simulink model "formation_planner_exp_cs_old"  (R2022b)
settings: Solver=ode5  StartTime=0.0  StopTime=80  FixedStep=1/1000  RelTol=1e-3
PreLoadFcn:
  | mbxruntime.callbacks.PreLoadFcn(bdroot);
PostLoadFcn:
  | mbxruntime.callbacks.PostLoadFcn(bdroot);
InitFcn:
  | mbxruntime.callbacks.InitFcn(bdroot);
StartFcn:
  | mbxruntime.callbacks.StartFcn(bdroot);
StopFcn:
  | mbxruntime.callbacks.StopFcn(bdroot);
model workspace (MAT data in the model file):
  mbox_table : object (value not decoded)
  model_closed = 0
  sim_status = 0
values from neighbouring files (symbols this model uses):
  c_factor = 43.75    [emplanner_init.m]
  car1_s = -10    [emplanner_init.m]
  car2_s = -20    [emplanner_init.m]
  cf = -175016    [emplanner_init.m]
  cr = -130634    [emplanner_init.m]
  KD_PID_distance = 0.0    (= 0)    [emplanner_init.m]
  KD_PID_speed = 0    [emplanner_init.m]
  KI_PID_distance = 0.0    (= 0)    [emplanner_init.m]
  KI_PID_speed = 0    [emplanner_init.m]
  KP_PID_distance = 0.5    [emplanner_init.m]
  KP_PID_speed = 1.8    [emplanner_init.m]
  la = 1.265    [emplanner_init.m]
  lb = 2.947-1.265    (= 1.682)    [emplanner_init.m]
  leader_global_kappa = global_kappa    [kappa.m]    (also in leader_global_path.mat = [0 0 0 0 0 0 0 0 0 0 0 0 ... (801 elements, 801x1)])
  leader_global_path_x = x_orgin.Data    [kappa.m]    (also in leader_global_path.mat = [2.22044604925e-16 0.999382255067 1.99750536558 2.9943522493)
  leader_global_path_y = y.Data    [kappa.m]    (also in leader_global_path.mat = [2 2 2 2 2 2 2 2 2 2 2 2 ... (801 elements, 801x1)])
  leader_global_yaw = yaw.Data    [kappa.m]    (also in leader_global_path.mat = [0 0 0 0 0 0 0 0 0 0 0 0 ... (801 elements, 801x1)])
  LQR_K1 = k(:,1)'    [emplanner_init.m]
  LQR_K2 = k(:,2)'    [emplanner_init.m]
  LQR_K3 = k(:,3)'    [emplanner_init.m]
  LQR_K4 = k(:,4)'    [emplanner_init.m]
  m = 2020    [emplanner_init.m]
  rack_displacement = [-39.14 , -37.2 , -35.29 , -33.43 , -31.6 , -29.81 , -28.06 , -26.34 , -24.66 ,      -23.01 , -21.38 , -19.79 , -18.23 , -16.69 , -15.18 , -13.7 , -12.23 , -10.8 , -9.38 , -7.98 ,     -6.61 , -5.25 , -3.91 , -2.59 , -1.29 , 0 , 1.27 , 2.54 , 3.78 , 5.02 , 6.24 , 7.46 , 8.66 ,      9.86 , 11.05 , 12.24 , 13.41 , 14.59 , 15.76 , 16.92 , 18.09 , 19.25 , 20.42 , 21.59 , 22.76 ,      23.93 , 25.11 , 26 ...(+26 chars)    [emplanner_init.m]
  right_wheel_ground = [-70 ,-67.2 , -64.4 , -61.6 , -58.8 , -56 , -53.2 , -50.4 , -47.6 , -44.8 , -42 ,      -39.2 , -36.4 , -33.6 , -30.8 , -28 , -25.2 , -22.4 , -19.6 , -16.8 , -14 , -11.2 , -8.4 , -5.6 ,      -2.8 , 0 , 2.8 , 5.6 , 8.4 , 11.2 , 14 , 16.8 , 19.6 , 22.4 , 25.2 , 28 , 30.8 , 33.6 , 36.4 ,      39.2 , 42 , 44.8 , 47.6 , 50.4 , 53.2 , 56 , 58.8 , 61.6 , 64.4 , 67.2 , 70 ]    [emplanner_init.m]
  vx_break_point = zeros(1,5000)    [emplanner_init.m]
undefined symbols (not defined in the file or in its folder): aubr, car1_global_kappa, car1_global_path_x, car1_global_path_y, car1_global_yaw, car2_global_kappa, car2_global_path_x, car2_global_path_y, car2_global_yaw, DiscIntNeverNeededParam, tablebr, vubr, warningInitialVelocity, x0
libraries: PreScanSimulinkLibrary x65, simulink x19, simulink_extras x14, Solver_SF x2
(part 10 of 31)

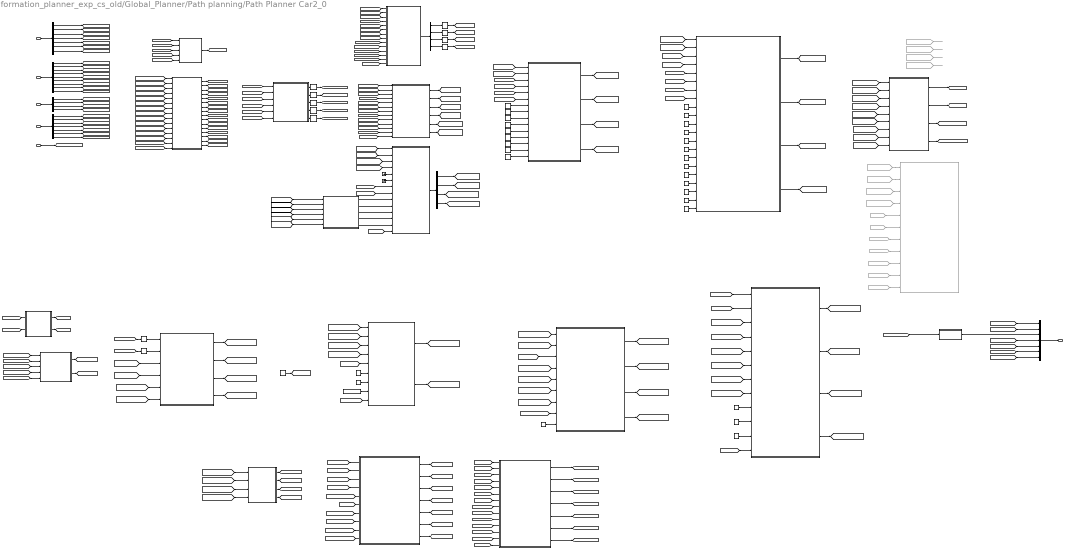
== system formation_planner_exp_cs_old/Global_Planner/Path planning/Path Planner Car2_0 ==
  referenceline info : Inport
  location info : Inport  Port=2
  perception info : Inport  Port=3
  pre_planning info : Inport  Port=4
  current time : Inport  Port=5
  Bus Creator : BusCreator  Inputs=7
  Bus Selector : BusSelector  OutputSignals=referenceline_x,referenceline_y,referenceline_heading,referenceline_kappa,origin_match_point_index,origin_x,origin_y
  Bus Selector1 : BusSelector  OutputSignals=host_x,host_y,host_heading_xy,host_vx,host_vy,host_yawrate,host_speed,host_ax,host_ay
  Bus Selector2 : BusSelector  OutputSignals=obs_x_set_gcs,obs_y_set_gcs,obs_velocity_set_gcs,obs_heading_set_gcs
  Bus Selector3 : BusSelector  OutputSignals=trajectory_x_gcs,trajectory_y_gcs,trajectory_heading_gcs,trajectory_kappa_gcs,trajectory_speed_gcs,trajectory_accel_gcs,trajectory_time_gcs
  Bus Selector4 : BusSelector  OutputSignals=s_set,l_set,dl_set,ddl_set
  Bus Selector5 : BusSelector  OutputSignals=s_set,l_set,s_dot_set,l_dot_set
  Cartesian2Frenet : Subsystem
  Cartesian2Frenet1 : Subsystem
  Constant : Constant  Value=1e6
  Constant1 : Constant  Value=2000
  Constant10 : Constant  Value=0.1
  Constant11 : Constant  Value=0.02
  Constant12 : Constant  Value=5
  Constant13 : Constant  Value=25000
  Constant14 : Constant  Value=50
  Constant15 : Constant  Value=20
  Constant16 : Constant  Value=50
  Constant{7,17..19} (4 alike) : Constant  Value=15
  Constant2 : Constant  Value=2
  Constant20 : Constant  Value=3
  Constant21 : Constant  Value=3
  Constant22 : Constant  Value=1.63
  Constant23 : Constant  Value=11
  Constant24 : Constant  Value=4000
  Constant25 : Constant  Value=100
  Constant26 : Constant  Value=10000000
  Constant27 : Constant  Value=0.2*9.8
  Constant28 : Constant  Value=50
  Constant29 : Constant  Value=500
  Constant3 : Constant  Value=3
  Constant4 : Constant  Value=10
  Constant5 : Constant  Value=11
  Constant6 : Constant  Value=4
  Constant8 : Constant
  Constant9 : Constant  Value=10
  Delay : Delay  DelayLength=1
  Delay1 : Delay  DelayLength=1
  Frenet2Cartesian task : MATLAB Function  TreatAsAtomicUnit=on
  From103 : From  Commented=on  GotoTag=dp_path_s_final
  From109 : From  Commented=on  GotoTag=dp_path_l_final
  From116 : From  Commented=on  GotoTag=dp_path_dl_final
  From117 : From  Commented=on  GotoTag=dp_path_ddl_final
  From120 : From  Commented=on  GotoTag=dp_path_s_final
  From124 : From  Commented=on  GotoTag=dp_path_l_final
  From125 : From  Commented=on  GotoTag=l_min
  From126 : From  Commented=on  GotoTag=l_max
  From129 : From  Commented=on  GotoTag=plan_start_l
  From130 : From  Commented=on  GotoTag=plan_start_dl
  From131 : From  Commented=on  GotoTag=plan_start_s
  From132 : From  Commented=on  GotoTag=static_obs_s_set
  From133 : From  Commented=on  GotoTag=static_obs_l_set
  From91 : From  Commented=on  GotoTag=qp_path_s_final
  From92 : From  Commented=on  GotoTag=qp_path_l_final
  Ground : Ground
  Ground1 : Ground
  MATLAB Function : MATLAB Function  TreatAsAtomicUnit=on
  MATLAB Function1 : MATLAB Function  TreatAsAtomicUnit=on
  MATLAB Function2 : MATLAB Function  TreatAsAtomicUnit=on
  Selector{1..9} (9 alike) : Selector  InputPortWidth=128  IndexOptions=Index vector (dialog)  Indices=1  OutputSizes=1
  calc path length and map between point and s1 : MATLAB Function  TreatAsAtomicUnit=on
  calc plan start info and stitch trajectory : MATLAB Function  TreatAsAtomicUnit=on
  calc speed planning start condition : MATLAB Function  TreatAsAtomicUnit=on
  generate convex space : MATLAB Function  TreatAsAtomicUnit=on
  generate st graph : MATLAB Function  TreatAsAtomicUnit=on
  genrate index to s : MATLAB Function  TreatAsAtomicUnit=on
  increase st point count : MATLAB Function  TreatAsAtomicUnit=on
  obs : Subsystem
  path and speed merge : MATLAB Function  TreatAsAtomicUnit=on
  path decision task : Subsystem
  path planning task : Subsystem
  plot : MATLAB Function  Commented=on  TreatAsAtomicUnit=on
  speed decision with dynamic planning(dp) : MATLAB Function  TreatAsAtomicUnit=on
  speed planning with quadratic programming (qp) : MATLAB Function  TreatAsAtomicUnit=on
  stitch trajectory : MATLAB Function  TreatAsAtomicUnit=on
  EM Planner result : Outport
  wires:
  referenceline info/1 -> Bus Selector/1
  location info/1 -> Bus Selector1/1
  perception info/1 -> Bus Selector2/1
  pre_planning info/1 -> Bus Selector3/1
  current time/1 -> [current_time]
  Bus Selector3/1 -> [pre_trajectory_x_gcs]  "<trajectory_x_gcs>"
  Bus Selector3/2 -> [pre_trajectory_y_gcs]  "<trajectory_y_gcs>"
  Bus Selector3/3 -> [pre_trajectory_heading_gcs]  "<trajectory_heading_gcs>"
  Bus Selector3/4 -> [pre_trajectory_kappa_gcs]  "<trajectory_kappa_gcs>"
  Bus Selector3/5 -> [pre_trajectory_speed_gcs]  "<trajectory_speed_gcs>"
  Bus Selector3/6 -> [pre_trajectory_accel_gcs]  "<trajectory_accel_gcs>"
  Bus Selector3/7 -> [pre_trajectory_time]  "<trajectory_time_gcs>"
  Bus Selector2/1 -> [obs_x_set_gcs]  "<obs_x_set_gcs>"
  Bus Selector2/2 -> [obs_y_set_gcs]  "<obs_y_set_gcs>"
  Bus Selector2/3 -> [obs_velocity_set_gcs]  "<obs_velocity_set_gcs>"
  Bus Selector2/4 -> [obs_heading_set_gcs]  "<obs_heading_set_gcs>"
  Bus Selector1/1 -> [host_x]  "<host_x>"
  Bus Selector1/2 -> [host_y]  "<host_y>"
  Bus Selector1/3 -> [host_heading_xy]  "<host_heading_xy>"
  Bus Selector1/4 -> [host_vx_vcs]  "<host_vx>"
  Bus Selector1/5 -> [host_vy_vcs]  "<host_vy>"
  Bus Selector1/6 -> [host_yawrate]  "<host_yawrate>"
  Bus Selector1/7 -> [host_speed]  "<host_speed>"
  Bus Selector1/8 -> [host_ax_vcs]  "<host_ax>"
  Bus Selector1/9 -> [host_ay_vcs]  "<host_ay>"
  Bus Selector/1 -> [referenceline_x]  "<referenceline_x>"
  Bus Selector/2 -> [referenceline_y]  "<referenceline_y>"
  Bus Selector/3 -> [referenceline_heading]  "<referenceline_heading>"
  Bus Selector/4 -> [referenceline_kappa]  "<referenceline_kappa>"
  [host_ay_vcs] -> calc plan start info and stitch trajectory/15(host_ay)
  [host_ax_vcs] -> calc plan start info and stitch trajectory/14(host_ax)
  [host_vy_vcs] -> calc plan start info and stitch trajectory/13(host_vy)
  [host_vx_vcs] -> calc plan start info and stitch trajectory/12(host_vx)
  [host_heading_xy] -> calc plan start info and stitch trajectory/11(host_heading_xy)
  [host_y] -> calc plan start info and stitch trajectory/10(host_y)
  [host_x] -> calc plan start info and stitch trajectory/9(host_x)
  [current_time] -> calc plan start info and stitch trajectory/8(current_time)
  [pre_trajectory_x_gcs] -> calc plan start info and stitch trajectory/1(pre_trajectory_x)
  [pre_trajectory_y_gcs] -> calc plan start info and stitch trajectory/2(pre_trajectory_y)
  [pre_trajectory_time] -> calc plan start info and stitch trajectory/7(pre_trajectory_time)
  [pre_trajectory_accel_gcs] -> calc plan start info and stitch trajectory/6(pre_trajectory_accel)
  [pre_trajectory_speed_gcs] -> calc plan start info and stitch trajectory/5(pre_trajectory_velocity)
  [pre_trajectory_kappa_gcs] -> calc plan start info and stitch trajectory/4(pre_trajectory_kappa)
  [pre_trajectory_heading_gcs] -> calc plan start info and stitch trajectory/3(pre_trajectory_heading)
  calc plan start info and stitch trajectory/1(plan_start_x) -> [plan_start_x_gcs]
  calc plan start info and stitch trajectory/2(plan_start_y) -> [plan_start_y_gcs]
  calc plan start info and stitch trajectory/3(plan_start_heading) -> [plan_start_heading_gcs]
  calc plan start info and stitch trajectory/4(plan_start_kappa) -> [plan_start_kappa_gcs]
  calc plan start info and stitch trajectory/5(plan_start_vx) -> [plan_start_vx_gcs]
  calc plan start info and stitch trajectory/6(plan_start_vy) -> [plan_start_vy_gcs]
  calc plan start info and stitch trajectory/7(plan_start_ax) -> [plan_start_ax_gcs]
  calc plan start info and stitch trajectory/8(plan_start_ay) -> [plan_start_ay_gcs]
  calc plan start info and stitch trajectory/9(plan_start_time) -> [plan_start_time]
  calc plan start info and stitch trajectory/10(stitch_x) -> [stitch_x_gcs]
  calc plan start info and stitch trajectory/11(stitch_y) -> [stitch_y_gcs]
  calc plan start info and stitch trajectory/12(stitch_heading) -> [stitch_heading_gcs]
  calc plan start info and stitch trajectory/13(stitch_kappa) -> [stitch_kappa_gcs]
  calc plan start info and stitch trajectory/14(stitch_speed) -> [stitch_speed_gcs]
  calc plan start info and stitch trajectory/15(stitch_accel) -> [stitch_accel_gcs]
  calc plan start info and stitch trajectory/16(stitch_time) -> [stitch_time]
  Bus Selector/5 -> [origin_match_point_index]  "<origin_match_point_index>"
  Bus Selector/6 -> [origin_x]  "<origin_x>"
  Bus Selector/7 -> [origin_y]  "<origin_y>"
  [referenceline_x] -> genrate index to s/1(path_x)
  [referenceline_y] -> genrate index to s/2(path_y)
  [origin_x] -> genrate index to s/3(origin_x)
  [origin_y] -> genrate index to s/4(origin_y)
  [origin_match_point_index] -> genrate index to s/5(origin_match_point_index)
  genrate index to s/1(index2s) -> [index2s]
  MATLAB Function2/5(proj_kappa_set) -> Selector5/1
  MATLAB Function2/3(proj_y_set) -> Selector3/1
  MATLAB Function2/1(match_point_index_set) -> Selector1/1
  MATLAB Function2/4(proj_heading_set) -> Selector4/1
  MATLAB Function2/2(proj_x_set) -> Selector2/1
  [plan_start_x_gcs] -> MATLAB Function2/1(x_set)
  [plan_start_y_gcs] -> MATLAB Function2/2(y_set)
  [referenceline_x] -> MATLAB Function2/3(frenet_path_x)
  [referenceline_y] -> MATLAB Function2/4(frenet_path_y)
  [referenceline_heading] -> MATLAB Function2/5(frenet_path_heading)
  [referenceline_kappa] -> MATLAB Function2/6(frenet_path_kappa)
  Selector1/1 -> [plan_start_match_point_index]
  Selector2/1 -> [plan_start_proj_x]
  Selector3/1 -> [plan_start_proj_y]
  Selector4/1 -> [plan_start_proj_heading]
  Selector5/1 -> [plan_start_proj_kappa]
  [plan_start_y_gcs] -> Cartesian2Frenet/2(y_set)
  [plan_start_x_gcs] -> Cartesian2Frenet/1(x_set)
  [plan_start_vx_gcs] -> Cartesian2Frenet/3(vx_set)
  [plan_start_vy_gcs] -> Cartesian2Frenet/4(vy_set)
  [plan_start_ax_gcs] -> Cartesian2Frenet/5(ax_set)
  [plan_start_ay_gcs] -> Cartesian2Frenet/6(ay_set)
  [referenceline_x] -> Cartesian2Frenet/7(frenet_path_x)
  [referenceline_y] -> Cartesian2Frenet/8(frenet_path_y)
  [plan_start_match_point_index] -> Cartesian2Frenet/9(proj_match_point_index_set)
  [plan_start_proj_x] -> Cartesian2Frenet/10(proj_x_set)
  [plan_start_proj_y] -> Cartesian2Frenet/11(proj_y_set)
  [plan_start_proj_heading] -> Cartesian2Frenet/12(proj_heading_set)
  [plan_start_proj_kappa] -> Cartesian2Frenet/13(proj_kappa_set)
  Cartesian2Frenet/1(Cartesian2FrenetOut) -> Bus Selector4/1
  Bus Selector4/4 -> Selector9/1  "<ddl_set>"
  Bus Selector4/3 -> Selector8/1  "<dl_set>"
  Bus Selector4/2 -> Selector7/1  "<l_set>"
  Bus Selector4/1 -> Selector6/1  "<s_set>"
  Selector6/1 -> [plan_start_s]
  Selector7/1 -> [plan_start_l]
  Selector8/1 -> [plan_start_dl]
  Selector9/1 -> [plan_start_ddl]
  [index2s] -> Cartesian2Frenet/14(index2s)
  Bus Creator/1 -> EM Planner result/1
  [trajectory_x_final] -> Bus Creator/1  "trajectory_x_gcs"
  [trajectory_time_final] -> Bus Creator/7  "trajectory_time_gcs"
  [trajectory_accel_final] -> Bus Creator/6  "trajectory_accel_gcs"
  [trajectory_speed_final] -> Bus Creator/5  "trajectory_speed_gcs"
  [trajectory_heading_final] -> MATLAB Function/1(trajectory_heading_final)
  [trajectory_kappa_final] -> Bus Creator/4  "trajectory_kappa_gcs"
  [trajectory_y_final] -> Bus Creator/2  "trajectory_y_gcs"
  [index2s] -> Frenet2Cartesian task/9(index2s)
  [referenceline_x] -> Frenet2Cartesian task/5(frenet_path_x)
  [referenceline_y] -> Frenet2Cartesian task/6(frenet_path_y)
  [referenceline_heading] -> Frenet2Cartesian task/7(frenet_path_heading)
  [referenceline_kappa] -> Frenet2Cartesian task/8(frenet_path_kappa)
  Frenet2Cartesian task/1(x_set) -> [trajectory_x_init]
  Frenet2Cartesian task/2(y_set) -> [trajectory_y_init]
  Frenet2Cartesian task/3(heading_set) -> [trajectory_heading_init]
  Frenet2Cartesian task/4(kappa_set) -> [trajectory_kappa_init]
  From120/1 -> plot/1(dp_s)
  From124/1 -> plot/2(dp_l)
  From125/1 -> plot/5(l_min)
  From126/1 -> plot/6(l_max)
  From130/1 -> plot/11(start_dl)
  From129/1 -> plot/10(start_l)
  From131/1 -> plot/9(start_s)
  From132/1 -> plot/7(obs_s_set)
  From133/1 -> plot/8(obs_l_set)
  path decision task/1(dp_path_s_final) -> [dp_path_s_final]
  path decision task/2(dp_path_l_final) -> [dp_path_l_final]
  path decision task/3(dp_path_dl_final) -> [dp_path_dl_final]
  path decision task/4(dp_path_ddl_final) -> [dp_path_ddl_final]
  [static_obs_s_set] -> path decision task/1(static_obs_s_set)
  [static_obs_l_set] -> path decision task/2(static_obs_l_set)
  [plan_start_ddl] -> path decision task/6(plan_start_ddl)
  [plan_start_dl] -> path decision task/5(plan_start_dl)
  [plan_start_l] -> path decision task/4(plan_start_l)
  [plan_start_s] -> path decision task/3(plan_start_s)
  [dp_path_s_final] -> path planning task/1(dp_path_s_final)
  [dp_path_l_final] -> path planning task/2(dp_path_l_final)
  [plan_start_l] -> path planning task/6(plan_start_l)
  [plan_start_ddl] -> path planning task/8(plan_start_ddl)
  [plan_start_dl] -> path planning task/7(plan_start_dl)
  Constant22/1 -> path planning task/19(host_w)
  Constant21/1 -> path planning task/18(host_d2)
  Constant20/1 -> path planning task/17(host_d1)
  Constant19/1 -> path planning task/16(qp_cost_end_ddl)
  Constant18/1 -> path planning task/15(qp_cost_end_dl)
  Constant17/1 -> path planning task/14(qp_cost_endl)
  Constant16/1 -> path planning task/13(qp_cost_centre)
  Constant15/1 -> path planning task/12(qp_cost_dddl)
  Constant14/1 -> path planning task/11(qp_cost_ddl)
  Constant13/1 -> path planning task/10(qp_cost_dl)
  Constant12/1 -> path planning task/9(qp_cost_l)
  Constant8/1 -> path decision task/15(dp_sample_l)
  Constant7/1 -> path decision task/14(dp_sample_s)
  Constant6/1 -> path decision task/13(dp_col)
  Constant5/1 -> path decision task/12(dp_row)
  Constant4/1 -> path decision task/11(dp_cost_ref)
  Constant3/1 -> path decision task/10(dp_cost_dddl)
  Constant/1 -> path decision task/7(dp_cost_collision)
  Constant1/1 -> path decision task/8(dp_cost_dl)
  Constant2/1 -> path decision task/9(dp_cost_ddl)
  [static_obs_s_set] -> path planning task/3(static_obs_s_set)
  [static_obs_l_set] -> path planning task/4(static_obs_l_set)
  Constant10/1 -> path planning task/20(delta_dl_max)
  Constant11/1 -> path planning task/21(delta_ddl_max)
  path planning task/1(qp_path_s_final) -> [qp_path_s_final]
  path planning task/2(qp_path_l_final) -> [qp_path_l_final]
  path planning task/3(qp_path_dl_final) -> [qp_path_dl_final]
  path planning task/4(qp_path_ddl_final) -> [qp_path_ddl_final]
  From91/1 -> plot/3(qp_s)
  From92/1 -> plot/4(qp_l)
  [plan_start_s] -> path planning task/5(plan_start_s)
  MATLAB Function/1(y) -> Bus Creator/3  "trajectory_heading_gcs"
  [obs_velocity_set_gcs] -> obs/7(obs_velocity_set_gcs)
  obs/6(dynamic_obs_vy_set) -> [dynamic_obs_vy_set]
  obs/3(dynamic_obs_x_set) -> [dynamic_obs_x_set]
  obs/5(dynamic_obs_vx_set) -> [dynamic_obs_vx_set]
  obs/4(dynamic_obs_y_set) -> [dynamic_obs_y_set]
  obs/2(static_obs_l_set) -> [static_obs_l_set]
  [index2s] -> obs/13(index2s)
  [referenceline_y] -> obs/10(referenceline_y)
  [host_heading_xy] -> obs/3(host_heading_xy)
  [obs_heading_set_gcs] -> obs/8(obs_heading_set_gcs)
  [referenceline_x] -> obs/9(referenceline_x)
  [referenceline_heading] -> obs/11(referenceline_heading)
  [referenceline_kappa] -> obs/12(referenceline_kappa)
  [host_y] -> obs/2(host_y)
  [host_x] -> obs/1(host_x)
  [obs_y_set_gcs] -> obs/6(obs_y_set_gcs)
  obs/1(static_obs_s_set) -> [static_obs_s_set]
  [obs_x_set_gcs] -> obs/5(obs_x_set_gcs)
  [trajectory_x_init] -> calc path length and map between point and s1/1(trajectory_x)
  calc path length and map between point and s1/2(path_index2s) -> [path_index2s]
  [trajectory_y_init] -> calc path length and map between point and s1/2(trajectory_y)
  calc path length and map between point and s1/1(path_s_end) -> [path_s_end]
  Bus Selector5/1 -> [dynamic_obs_s_set]  "<s_set>"
  [trajectory_x_init] -> MATLAB Function1/3(frenet_path_x)
  MATLAB Function1/5(proj_kappa_set) -> Cartesian2Frenet1/13(proj_kappa_set)
  [dynamic_obs_x_set] -> MATLAB Function1/1(x_set)
  Ground1/1 -> Cartesian2Frenet1/6(ay_set)
  MATLAB Function1/4(proj_heading_set) -> Cartesian2Frenet1/12(proj_heading_set)
  MATLAB Function1/2(proj_x_set) -> Cartesian2Frenet1/10(proj_x_set)
  [trajectory_y_init] -> MATLAB Function1/4(frenet_path_y)
  [dynamic_obs_vx_set] -> Cartesian2Frenet1/3(vx_set)
  [dynamic_obs_y_set] -> Cartesian2Frenet1/2(y_set)
  [dynamic_obs_vy_set] -> Cartesian2Frenet1/4(vy_set)
  MATLAB Function1/3(proj_y_set) -> Cartesian2Frenet1/11(proj_y_set)
  Cartesian2Frenet1/1(Cartesian2FrenetOut) -> Bus Selector5/1
  [trajectory_x_init] -> Cartesian2Frenet1/7(frenet_path_x)
  [path_index2s] -> Cartesian2Frenet1/14(index2s)
  Ground/1 -> Cartesian2Frenet1/5(ax_set)
  [trajectory_kappa_init] -> MATLAB Function1/6(frenet_path_kappa)
  MATLAB Function1/1(match_point_index_set) -> Cartesian2Frenet1/9(proj_match_point_index_set)
  Bus Selector5/2 -> [dynamic_obs_l_set]  "<l_set>"
  [trajectory_y_init] -> Cartesian2Frenet1/8(frenet_path_y)
  [dynamic_obs_y_set] -> MATLAB Function1/2(y_set)
  [trajectory_heading_init] -> MATLAB Function1/5(frenet_path_heading)
  Bus Selector5/3 -> [dynamic_obs_s_dot_set]  "<s_dot_set>"
  [dynamic_obs_x_set] -> Cartesian2Frenet1/1(x_set)
  Bus Selector5/4 -> [dynamic_obs_l_dot_set]  "<l_dot_set>"
  [dp_speed_t] -> generate convex space/2(dp_speed_t)
  increase st point count/4(relative_time) -> [relative_time]
  [dp_speed_s] -> generate convex space/1(dp_speed_s)
  [dynamic_obs_l_set] -> generate st graph/4(dynamic_obs_l_set)
  increase st point count/2(s_dot) -> [s_dot]
  stitch trajectory/5(trajectory_speed_final) -> [trajectory_speed_final]
  [path_index2s] -> generate convex space/3(path_index2s)
  increase st point count/3(s_dot2) -> [s_dot2]
  [dynamic_obs_s_set] -> generate st graph/3(dynamic_obs_s_set)
  Delay/1 -> generate st graph/1(pre_trajectory_s)
  stitch trajectory/7(trajectory_time_final) -> [trajectory_time_final]
  Delay1/1 -> generate st graph/2(pre_trajectory_t)
  generate st graph/4(obs_st_t_out_set) -> [obs_st_t_out_set]
  Constant24/1 -> speed decision with dynamic planning(dp)/6(w_cost_ref_speed)
  path and speed merge/6(trajectory_accel) -> [trajectory_accel]
  [trajectory_x] -> stitch trajectory/1(trajectory_x)
  [relative_time] -> path and speed merge/4(relative_time)
  calc speed planning start condition/2(plan_start_s_dot2) -> [plan_start_s_dot2]
  [trajectory_x_init] -> path and speed merge/7(trajectory_x_init)
  [s_dot2] -> path and speed merge/3(s_dot2)
  [s_dot] -> path and speed merge/2(s_dot)
  increase st point count/1(s) -> [s]
  [s] -> path and speed merge/1(s)
  [plan_start_vy_gcs] -> calc speed planning start condition/2(plan_start_vy)
  stitch trajectory/3(trajectory_heading_final) -> [trajectory_heading_final]
  [plan_start_vx_gcs] -> calc speed planning start condition/1(plan_start_vx)
  [obs_st_t_in_set] -> generate convex space/6(obs_st_t_in_set)
  [obs_st_t_out_set] -> generate convex space/7(obs_st_t_out_set)
  [obs_st_s_out_set] -> generate convex space/5(obs_st_s_out_set)
  [trajectory_kappa_init] -> generate convex space/8(trajectory_kappa_init)
  generate convex space/2(s_ub) -> [s_ub]
  [plan_start_s_dot] -> speed decision with dynamic planning(dp)/9(plan_start_s_dot)
  [qp_s_dot_init] -> increase st point count/2(s_dot_init)
  [dynamic_obs_s_dot_set] -> generate st graph/5(dynamic_obs_s_dot_set)
  path and speed merge/4(trajectory_kappa) -> [trajectory_kappa]
  speed planning with quadratic programming (qp)/3(qp_s_dot2_init) -> [qp_s_dot2_init]
  [reference_speed] -> speed planning with quadratic programming (qp)/12(speed_reference)
  calc speed planning start condition/1(plan_start_s_dot) -> [plan_start_s_dot]
  Constant28/1 -> speed planning with quadratic programming (qp)/10(w_cost_v_ref)
  [obs_st_t_in_set] -> speed decision with dynamic planning(dp)/3(obs_st_t_in_set)
  [s_dot_ub] -> speed planning with quadratic programming (qp)/8(s_dot_ub)
  [dynamic_obs_l_dot_set] -> generate st graph/6(dynamic_obs_l_dot_set)
  stitch trajectory/2(trajectory_y_final) -> [trajectory_y_final]
  [relative_time] -> Delay1/1
  speed planning with quadratic programming (qp)/1(qp_s_init) -> [qp_s_init]
  generate st graph/3(obs_st_t_in_set) -> [obs_st_t_in_set]
  Constant9/1 -> speed planning with quadratic programming (qp)/9(w_cost_s_dot2)
  speed decision with dynamic planning(dp)/2(dp_speed_t) -> [dp_speed_t]
  generate st graph/2(obs_st_s_out_set) -> [obs_st_s_out_set]
  [stitch_x_gcs] -> stitch trajectory/8(stitch_x)
  Constant27/1 -> generate convex space/9(max_lateral_accel)
  [obs_st_s_out_set] -> speed decision with dynamic planning(dp)/2(obs_st_s_out_set)
  [plan_start_heading_gcs] -> calc speed planning start condition/5(plan_start_heading)
  Constant26/1 -> speed decision with dynamic planning(dp)/8(w_cost_obs)
  path and speed merge/7(trajectory_time) -> [trajectory_time]
  path and speed merge/5(trajectory_speed) -> [trajectory_speed]
  [qp_s_dot2_init] -> increase st point count/3(s_dot2_init)
  [path_index2s] -> path and speed merge/6(path_s)
  [trajectory_heading_init] -> path and speed merge/9(trajectory_heading_init)
  [s_lb] -> speed planning with quadratic programming (qp)/5(s_lb)
  [trajectory_y_init] -> path and speed merge/8(trajectory_y_init)
  [s_ub] -> speed planning with quadratic programming (qp)/6(s_ub)
  [plan_start_time] -> path and speed merge/5(current_time)
  [trajectory_time] -> stitch trajectory/7(trajectory_time)
  [obs_st_s_in_set] -> generate convex space/4(obs_st_s_in_set)
  [trajectory_kappa] -> stitch trajectory/4(trajectory_kappa)
  [plan_start_s_dot2] -> speed planning with quadratic programming (qp)/2(plan_start_s_dot2)
  path and speed merge/3(trajectory_heading) -> [trajectory_heading]
  [trajectory_kappa_init] -> path and speed merge/10(trajectory_kappa_init)
  generate convex space/1(s_lb) -> [s_lb]
  path and speed merge/2(trajectory_y) -> [trajectory_y]
  [trajectory_y] -> stitch trajectory/2(trajectory_y)
  generate convex space/4(s_dot_ub) -> [s_dot_ub]
  [obs_st_s_in_set] -> speed decision with dynamic planning(dp)/1(obs_st_s_in_set)
  [qp_s_init] -> increase st point count/1(s_init)
  [stitch_time] -> stitch trajectory/14(stitch_time)
  [stitch_kappa_gcs] -> stitch trajectory/11(stitch_kappa)
  [stitch_accel_gcs] -> stitch trajectory/13(stitch_accel)
  [stitch_heading_gcs] -> stitch trajectory/10(stitch_heading)
  stitch trajectory/1(trajectory_x_final) -> [trajectory_x_final]
  [plan_start_s_dot] -> speed planning with quadratic programming (qp)/1(plan_start_s_dot)
  [reference_speed] -> speed decision with dynamic planning(dp)/5(reference_speed_unlimit)
  speed planning with quadratic programming (qp)/2(qp_s_dot_init) -> [qp_s_dot_init]
  speed planning with quadratic programming (qp)/4(relative_time_init) -> [relative_time_init]
  stitch trajectory/4(trajectory_kappa_final) -> [trajectory_kappa_final]
  [trajectory_speed] -> stitch trajectory/5(trajectory_speed)
  [stitch_speed_gcs] -> stitch trajectory/12(stitch_speed)
  [plan_start_ax_gcs] -> calc speed planning start condition/3(plan_start_ax)
  [trajectory_accel] -> stitch trajectory/6(trajectory_accel)
  path and speed merge/1(trajectory_x) -> [trajectory_x]
  [relative_time_init] -> increase st point count/4(relative_time_init)
  [plan_start_ay_gcs] -> calc speed planning start condition/4(plan_start_ay)
  [trajectory_heading] -> stitch trajectory/3(trajectory_heading)
  [dp_speed_t] -> speed planning with quadratic programming (qp)/4(dp_speed_t)
  Constant23/1 -> [reference_speed]
  [obs_st_t_out_set] -> speed decision with dynamic planning(dp)/4(obs_st_t_out_set)
  speed decision with dynamic planning(dp)/1(dp_speed_s) -> [dp_speed_s]
  Constant25/1 -> speed decision with dynamic planning(dp)/7(w_cost_accel)
  [stitch_y_gcs] -> stitch trajectory/9(stitch_y)
  Constant29/1 -> speed planning with quadratic programming (qp)/11(w_cost_jerk)
  [dp_speed_s] -> speed planning with quadratic programming (qp)/3(dp_speed_s)
  [s] -> Delay/1
  generate st graph/1(obs_st_s_in_set) -> [obs_st_s_in_set]
  generate convex space/3(s_dot_lb) -> [s_dot_lb]
  [s_dot_lb] -> speed planning with quadratic programming (qp)/7(s_dot_lb)
  stitch trajectory/6(trajectory_accel_final) -> [trajectory_accel_final]
  [qp_path_ddl_final] -> Frenet2Cartesian task/4(ddl_set)
  [qp_path_l_final] -> Frenet2Cartesian task/2(l_set)
  [qp_path_s_final] -> Frenet2Cartesian task/1(s_set)
  [qp_path_dl_final] -> Frenet2Cartesian task/3(dl_set)
  From103/1 -> ?
  From117/1 -> ?
  From116/1 -> ?
  From109/1 -> ?
  [host_speed] -> obs/4(host_speed)
